simulink model "internship_linear_simple_model_v3"  (R2024a)
settings: Solver=ode3  StartTime=0.0  StopTime=19  FixedStep=0.01  RelTol=1e-3
InitFcn:
  | init_parameter;
values from neighbouring files (symbols this model uses):
  A = [-(Caf+Car)/(m*u0) (b*Car-a*Caf)/(m*u0)-u0 ... (first row only)    [init_parameter.m]
  B = [Caf/m; a*Caf/Iz]    [init_parameter.m]
  C = eye(2)    [init_parameter.m]
  D = [0; 0]    [init_parameter.m]
settings Model: Creator=Changsun Ahn  LastModifiedBy=xslee
settings SolverCC: AlgebraicLoopSolver=TrustRegion
settings DataIOCC: LimitDataPoints=on  SaveFormat=Array  SignalLoggingSaveFormat=ModelDataLogs  ReturnWorkspaceOutputs=off  SignalLoggingName=sigsOut
settings OptimizationCC: ExpressionDepthLimit=2147483647  LifeSpan=inf
settings DebuggingCC: SaveWithParameterizedLinksMsg=none  UnderspecifiedInitializationDetection=Classic  MergeDetectMultiDrivingBlocksExec=none  SignalResolutionControl=TryResolveAllWithWarning  MultiTaskDSMMsg=warning  MultiTaskCondExecSysMsg=none  UnconnectedInputMsg=warning  UnconnectedOutputMsg=warning  UnconnectedLineMsg=warning  StateNameClashWarn=warning  SFUnexpectedBacktrackingDiag=warning  SFNoUnconditionalDefaultTransitionDiag=warning  SFExecutionAtInitializationDiag=none  ArithmeticOperatorsInVariantConditions=warning
settings HardwareCC: ProdBitPerPointer=32  ProdBitPerSizeT=32  ProdBitPerPtrDiffT=32  ProdLargestAtomicFloat=None  ProdIntDivRoundTo=Undefined  ProdEndianess=Unspecified  ProdWordSize=32  ProdHWDeviceType=32-bit Generic  TargetBitPerPointer=64  TargetBitPerSizeT=64  TargetBitPerPtrDiffT=64  TargetLongLongMode=on  TargetIntDivRoundTo=Zero  TargetEndianess=LittleEndian  TargetWordSize=64  TargetHWDeviceType=MATLAB Host  ProdEqTarget=off
settings ModelReferenceCC: EnableRefExpFcnMdlSchedulingChecks=on  PropagateSignalLabelsOutOfModel=off
settings SFSimCC: SimUseLocalCustomCode=off  CustomCodeUndefinedFunction=UseInterfaceOnly
settings RTWCC: RTWUseLocalCustomCode=off  GPUComputeCapability=3.5  DLArmComputeVersion=19.05
settings CodeAppCC: StateflowObjectComments=on
settings GRTTargetCC: TargetLangStandard=C89/C90 (ANSI)  CombineOutputUpdateFcns=off  GRTInterface=on
settings ConfigComp: CovMetricSettings=dw  CovSaveCumulativeToWorkspaceVar=on  CovSaveSingleToWorkspaceVar=on  CovExternalEMLEnable=off

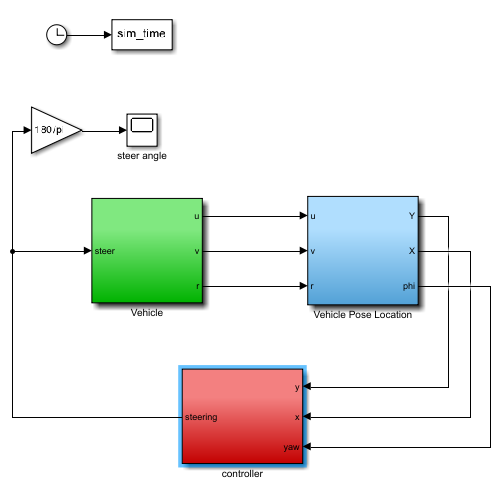
[thumbnail: Simulink's stored preview of the top-level diagram]
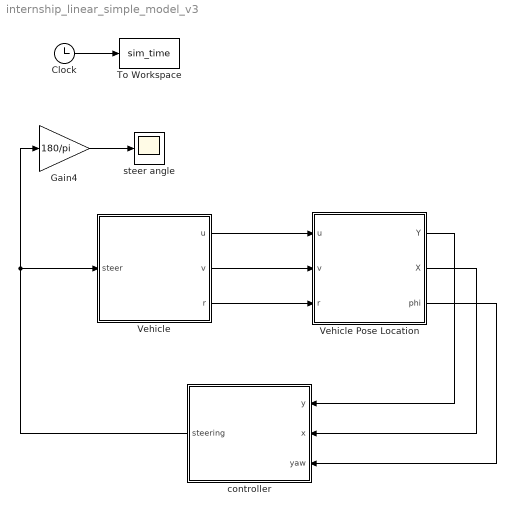
== system internship_linear_simple_model_v3 ==
  Clock : Clock
  Gain4 : Gain  Gain=180/pi
  To Workspace : ToWorkspace  VariableName=sim_time  SaveFormat=Timeseries  SampleTime=-1
  Vehicle : Subsystem
  Vehicle Pose Location : Subsystem
  controller : Subsystem
  steer angle : Scope
  wires:
  Vehicle/2(v) -> Vehicle Pose Location/2(v)
  Vehicle/3(r) -> Vehicle Pose Location/3(r)
  Vehicle Pose Location/1(Y) -> controller/1(y)
  Vehicle Pose Location/3(phi) -> controller/3(yaw)
  Vehicle Pose Location/2(X) -> controller/2(x)
  Vehicle/1(u) -> Vehicle Pose Location/1(u)
  Clock/1 -> To Workspace/1
  controller/1(steering) -> Vehicle/1(steer), Gain4/1
  Gain4/1 -> steer angle/1

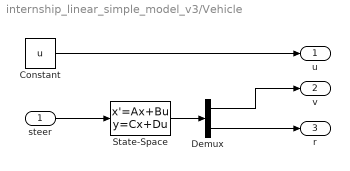
== system internship_linear_simple_model_v3/Vehicle ==
  steer : Inport
  Constant : Constant  Value=u
  Demux : Demux  Outputs=2
  State-Space : StateSpace  A=A  B=B  C=C  D=D  InitialCondition=[0;0]
  u : Outport
  v : Outport  Port=2
  r : Outport  Port=3
  wires:
  Constant/1 -> u/1
  State-Space/1 -> Demux/1
  steer/1 -> State-Space/1
  Demux/2 -> r/1
  Demux/1 -> v/1

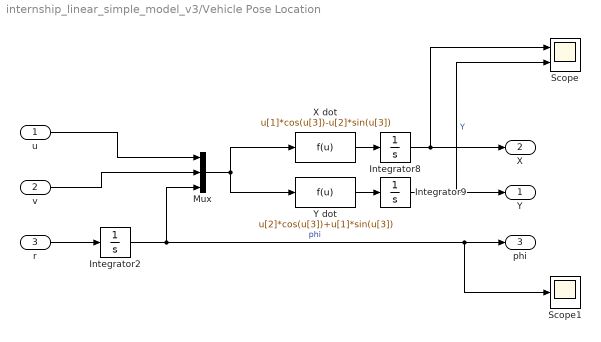
== system internship_linear_simple_model_v3/Vehicle Pose Location ==
  u : Inport
  v : Inport  Port=2
  r : Inport  Port=3
  Integrator2 : Integrator
  Integrator8 : Integrator
  Integrator9 : Integrator
  Mux : Mux  Inputs=3
  Scope : Scope  NumInputPorts=2
  Scope1 : Scope
  X dot : Fcn  Expr=u[1]*cos(u[3])-u[2]*sin(u[3])
  Y dot : Fcn  Expr=u[2]*cos(u[3])+u[1]*sin(u[3])
  Y : Outport
  X : Outport  Port=2
  phi : Outport  Port=3
  wires:
  Mux/1 -> Y dot/1, X dot/1
  Integrator9/1 -> Scope/2, Y/1  "Y"
  v/1 -> Mux/2
  Y dot/1 -> Integrator9/1
  u/1 -> Mux/1
  Integrator2/1 -> Scope1/1, phi/1, Mux/3  "phi"
  X dot/1 -> Integrator8/1
  Integrator8/1 -> Scope/1, X/1
  r/1 -> Integrator2/1

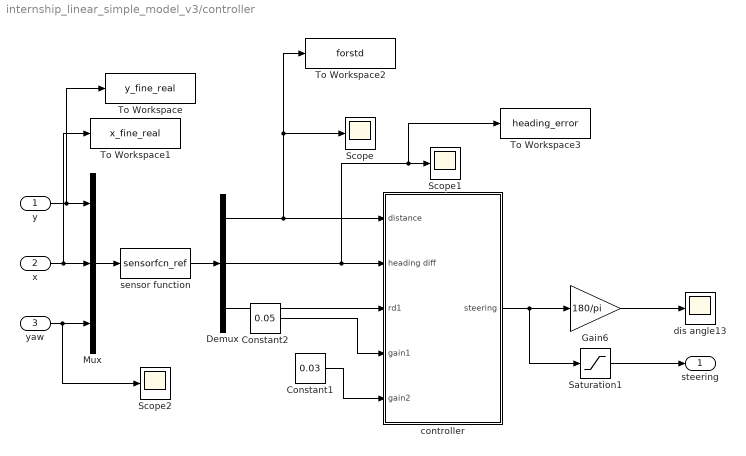
== system internship_linear_simple_model_v3/controller ==
  y : Inport
  x : Inport  Port=2
  yaw : Inport  Port=3
  Constant1 : Constant  Value=0.03
  Constant2 : Constant  Value=0.05
  Demux : Demux  Outputs=3
  Gain6 : Gain  Gain=180/pi
  Mux : Mux  Inputs=3
  Saturation1 : Saturate  UpperLimit=30*pi/180  LowerLimit=-30*pi/180
  Scope : Scope
  Scope1 : Scope
  Scope2 : Scope
  To Workspace : ToWorkspace  VariableName=y_fine_real  SaveFormat=Timeseries  SampleTime=-1
  To Workspace1 : ToWorkspace  VariableName=x_fine_real  SaveFormat=Timeseries  SampleTime=-1
  To Workspace2 : ToWorkspace  VariableName=forstd  SaveFormat=Timeseries  SampleTime=-1
  To Workspace3 : ToWorkspace  VariableName=heading_error  SaveFormat=Timeseries  SampleTime=-1
  controller : Subsystem
  dis angle13 : Scope
  sensor function : MATLABFcn  MATLABFcn=sensorfcn_ref
  steering : Outport
  wires:
  Constant2/1 -> controller/4(gain1)
  controller/1(steering) -> Gain6/1, Saturation1/1
  Gain6/1 -> dis angle13/1
  Saturation1/1 -> steering/1
  Constant1/1 -> controller/5(gain2)
  y/1 -> To Workspace/1, Mux/1
  x/1 -> To Workspace1/1, Mux/2
  Mux/1 -> sensor function/1
  yaw/1 -> Scope2/1, Mux/3
  Demux/1 -> Scope/1, To Workspace2/1, controller/1(distance)
  Demux/2 -> To Workspace3/1, Scope1/1, controller/2(heading diff)
  Demux/3 -> controller/3(rd1)
  sensor function/1 -> Demux/1

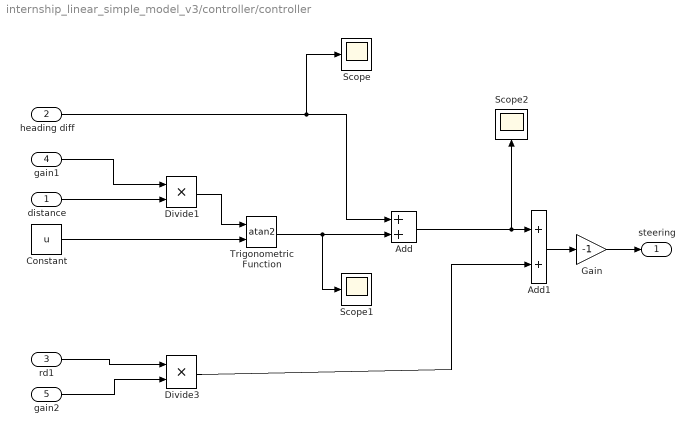
== system internship_linear_simple_model_v3/controller/controller ==
  distance : Inport
  heading diff : Inport  Port=2
  rd1 : Inport  Port=3
  gain1 : Inport  Port=4
  gain2 : Inport  Port=5
  Add : Sum
  Add1 : Sum
  Constant : Constant  Value=u
  Divide1 : Product  Inputs=**
  Divide3 : Product  Inputs=**
  Gain : Gain  Gain=-1
  Scope : Scope
  Scope1 : Scope
  Scope2 : Scope
  Trigonometric Function : Trigonometry  Operator=atan2
  steering : Outport
  wires:
  Divide3/1 -> Add1/2
  Add1/1 -> Gain/1
  gain1/1 -> Divide1/1
  distance/1 -> Divide1/2
  Add/1 -> Scope2/1, Add1/1
  Divide1/1 -> Trigonometric Function/1
  Constant/1 -> Trigonometric Function/2
  Trigonometric Function/1 -> Scope1/1, Add/2
  gain2/1 -> Divide3/2
  Gain/1 -> steering/1
  rd1/1 -> Divide3/1
  heading diff/1 -> Add/1, Scope/1
